simulink model "Q5"  (R2021b)
settings: Solver=VariableStepAuto  StartTime=0.0  StopTime=20  RelTol=1e-3
settings Model: Creator=DSDLn  LastModifiedBy=DSDLn

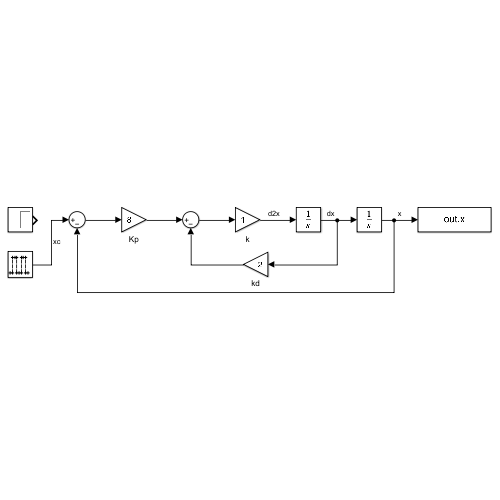
[thumbnail: Simulink's stored preview of the top-level diagram]
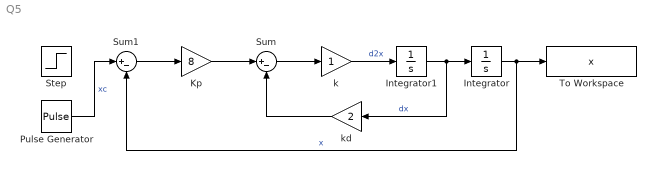
== system Q5 ==
  Integrator : Integrator
  Integrator1 : Integrator
  Kp : Gain  Gain=8
  Pulse Generator : DiscretePulseGenerator  Period=200  PulseWidth=100  SampleTime=0.1
  Step : Step  Time=0  SampleTime=0.1
  Sum : Sum  Inputs=|+-
  Sum1 : Sum  Inputs=|+-
  To Workspace : ToWorkspace  VariableName=x  SampleTime=-1
  k : Gain
  kd : Gain  Gain=2
  wires:
  Integrator/1 -> Sum1/2, To Workspace/1  "x"
  Integrator1/1 -> kd/1, Integrator/1  "dx"
  k/1 -> Integrator1/1  "d2x"
  Sum/1 -> k/1
  kd/1 -> Sum/2
  Kp/1 -> Sum/1
  Sum1/1 -> Kp/1
  Pulse Generator/1 -> Sum1/1  "xc"
